simulink library "plant3D"  (R2020a)
settings: Solver=VariableStepAuto  StartTime=0.0  StopTime=10.0  RelTol=1e-3
undefined symbols (not defined in the file): Env, PLANT, Veh
libraries: gravLoads3D_ul x1, motor3D_cl x1, sixDoFDynamics_cl x1
settings Model: Creator=John Jr  LastModifiedBy=John Jr

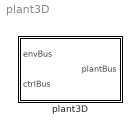
== system plant3D ==
  plant3D : Subsystem  VariantControl=strcmpi(PLANT,'wind3D')

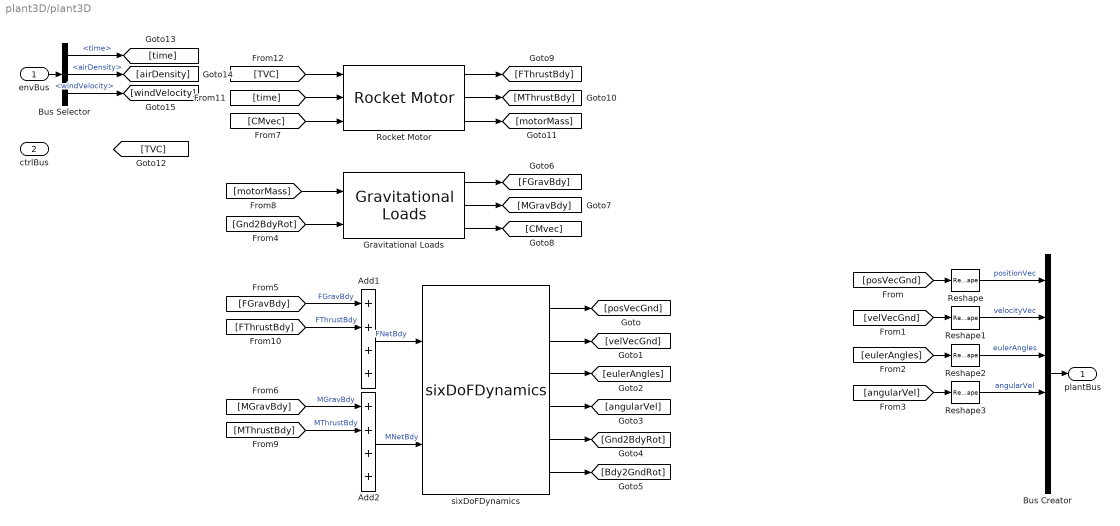
== system plant3D/plant3D ==
  envBus : Inport
  ctrlBus : Inport  Port=2
  Add1 : Sum  Inputs=++++
  Add2 : Sum  Inputs=++++
  Bus Creator : BusCreator  Inputs=6
  Bus Selector : BusSelector  OutputSignals=time,airDensity,windVelocity
  Gravitational Loads : gravLoads3D_ul/Gravitational Loads  g=Env.grav.Value  m=Veh.structMass.Value  CG1=Veh.rCMpad_B.Value  CG2=Veh.rCMair_B.Value  t_b=Veh.motor.burnTime.Value
  Reshape{,1..3} (4 alike) : Reshape  OutputDimensionality=Column vector (2-D)
  Rocket Motor : motor3D_cl/Rocket Motor  m_m=Veh.motor.motorMass.Value  m_f=Veh.motor.fuelMass.Value  t_b=Veh.motor.burnTime.Value  rM=Veh.motor.position.Value
  sixDoFDynamics : sixDoFDynamics_cl/sixDoFDynamics  vcl=vcl
  plantBus : Outport
  wires:
  Bus Selector/3 -> [windVelocity]  "<windVelocity>"
  Bus Selector/2 -> [airDensity]  "<airDensity>"
  Bus Selector/1 -> [time]  "<time>"
  envBus/1 -> Bus Selector/1
  sixDoFDynamics/1 -> [posVecGnd]
  sixDoFDynamics/2 -> [velVecGnd]
  sixDoFDynamics/6 -> [Bdy2GndRot]
  sixDoFDynamics/5 -> [Gnd2BdyRot]
  sixDoFDynamics/4 -> [angularVel]
  sixDoFDynamics/3 -> [eulerAngles]
  Bus Creator/1 -> plantBus/1
  Reshape/1 -> Bus Creator/1  "positionVec"
  Reshape1/1 -> Bus Creator/2  "velocityVec"
  Reshape2/1 -> Bus Creator/3  "eulerAngles"
  Reshape3/1 -> Bus Creator/4  "angularVel"
  [angularVel] -> Reshape3/1
  [eulerAngles] -> Reshape2/1
  [velVecGnd] -> Reshape1/1
  [posVecGnd] -> Reshape/1
  [Gnd2BdyRot] -> Gravitational Loads/2
  Gravitational Loads/1 -> [FGravBdy]
  Gravitational Loads/2 -> [MGravBdy]
  Gravitational Loads/3 -> [CMvec]
  Add1/1 -> sixDoFDynamics/1  "FNetBdy"
  Add2/1 -> sixDoFDynamics/2  "MNetBdy"
  [FGravBdy] -> Add1/1  "FGravBdy"
  [MGravBdy] -> Add2/1  "MGravBdy"
  [CMvec] -> Rocket Motor/3
  Rocket Motor/1 -> [FThrustBdy]
  Rocket Motor/2 -> [MThrustBdy]
  Rocket Motor/3 -> [motorMass]
  [motorMass] -> Gravitational Loads/1
  [MThrustBdy] -> Add2/2  "MThrustBdy"
  [FThrustBdy] -> Add1/2  "FThrustBdy"
  [TVC] -> Rocket Motor/1
  [time] -> Rocket Motor/2
